simulink model "trafficLight"  (R2024a)
settings: Solver=FixedStepDiscrete  StartTime=0.0  StopTime=inf  FixedStep=1e-2  RelTol=1e-3  EnableMultiTasking=on
libraries: stm32f4xxblockslib x4
settings Model: STM32="{\"DigitalPortWrite\":[{\"ID\":\"untitled:5\"},{\"ID\":\"untitled:6\"},{\"ID\":\"untitled:7\"},{\"ID\":\"trafficLight:5\"},{\"ID\":\"trafficLight:7\"},{\"ID\":\"trafficLight:6\"}],\"HardwareInterrupt\":[{\"ID\":\"untitled:8\"},{\"ID\":\"trafficLight:8\"}]}"  Creator=User  LastModifiedBy=User
settings SolverCC: AutoInsertRateTranBlk=on
settings OptimizationCC: EnhancedBackFolding=on  PassReuseOutputArgsAs=Individual arguments  ZeroExternalMemoryAtStartup=off  ZeroInternalMemoryAtStartup=off  MaxStackSize=64  OptimizeBlockOrder=speed  DifferentSizesBufferReuse=on  OptimizationCustomize=off  EfficientTunableParamExpr=on
settings DebuggingCC: MultiTaskDSMMsg=none  ParameterTunabilityLossMsg=error
settings HardwareCC: ProdBitPerPointer=32  ProdBitPerSizeT=32  ProdBitPerPtrDiffT=32  ProdLargestAtomicInteger=Long  ProdLargestAtomicFloat=Double  ProdWordSize=32  ProdLongLongMode=on  ProdHWDeviceType=ARM Compatible->ARM Cortex-M
settings SFSimCC: MATLABDynamicMemAlloc=off
settings RTWCC: Description=Embedded Coder  SystemTargetFile=ert.tlc  HardwareBoard=STM32F4xx Based  TemplateMakefile=ert_default_tmf  Toolchain=GNU Tools for ARM Embedded Processors
settings CodeAppCC: ForceParamTrailComments=on  IgnoreCustomStorageClasses=off  OperatorAnnotations=on  SimulinkDataObjDesc=on  SFDataObjDesc=on  InsertBlockDesc=on
settings ERTTargetCC: TargetLangStandard=C99 (ISO)  CodeReplacementLibrary=ARM Cortex-M  ExtModeTransport=3  ExtModeStaticAlloc=on  ExtModeStaticAllocSize=2048  ExtModeMexFile=ext_xcp  ExtModeIntrfLevel=Level2 - Open

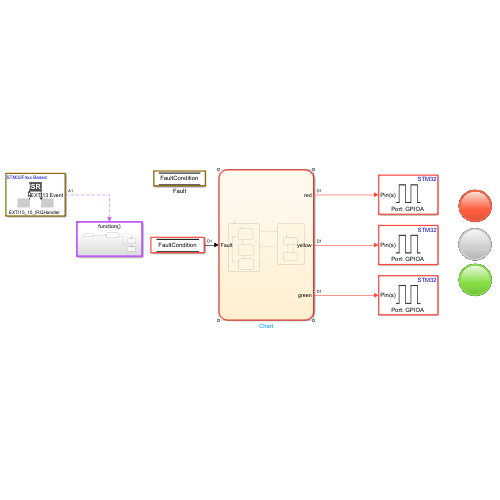
[thumbnail: Simulink's stored preview of the top-level diagram]
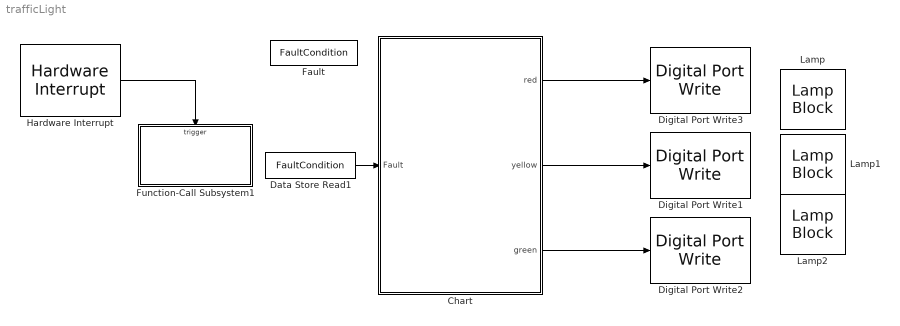
== system trafficLight ==
  Chart : Stateflow chart  TreatAsAtomicUnit=on
  Data Store Read1 : DataStoreRead  DataStoreName=FaultCondition  IndexOptions=Index vector (dialog)  Indices=1  OutputSizes=1
  Digital Port Write1 : stm32f4xxblockslib/Digital Port Write  PortName=GPIOA  PinNumber=[11]  ReadOperation=off  IOAsArray=on  EnableSimPort=off  hoistedMaskSrc=ECSoC/ECSimCodegen/Digital Port Write
  Digital Port Write2 : stm32f4xxblockslib/Digital Port Write  PortName=GPIOA  PinNumber=[12]  ReadOperation=off  IOAsArray=on  EnableSimPort=off  hoistedMaskSrc=ECSoC/ECSimCodegen/Digital Port Write
  Digital Port Write3 : stm32f4xxblockslib/Digital Port Write  PortName=GPIOA  PinNumber=[10]  ReadOperation=off  IOAsArray=on  EnableSimPort=off  hoistedMaskSrc=ECSoC/ECSimCodegen/Digital Port Write
  Fault : DataStoreMemory  DataStoreName=FaultCondition  WriteAfterWriteMsg=warning  ShowAdditionalParam=off
  Function-Call Subsystem1 : Subsystem  TreatAsAtomicUnit=on
  Hardware Interrupt : stm32f4xxblockslib/Hardware Interrupt  ISRGroup=External interrupts (EXTI)  ISRName=EXTI15_10_IRQHandler  ISRNumber=55  EventsList={ 'off', 'EXTI15 Event', '1'; 'off', 'EXTI14 Event', '2'; 'on', 'EXTI13 Event', '3'; 'off', 'EXTI12 Event', '4'; 'off', 'EXTI11 Event', '5'; 'off', 'EXTI10 Event', '6'; 'off', 'Custom event', '7' }  SelectedEvents={'EXTI13 Event'}  TaskPriority=30  DisablePreemption=on  ClearInterruptFlagsAtEndOfEvent=off  InterruptDefinitionFile=$(TARGET_ROOT)/registry/interrupts/STM32F4xxBased_interrupts.xml  HardwareBoard=STM32F4xx Based  EnableSimPort=off
  Lamp : LampBlock  LabelPosition=Hide
  Lamp1 : LampBlock  LabelPosition=Hide
  Lamp2 : LampBlock  LabelPosition=Hide
  wires:
  Chart/1(red) -> Digital Port Write3/1
  Chart/2(yellow) -> Digital Port Write1/1
  Chart/3(green) -> Digital Port Write2/1
  Hardware Interrupt/1 -> Function-Call Subsystem1/Trigger
  Data Store Read1/1 -> Chart/1(Fault)

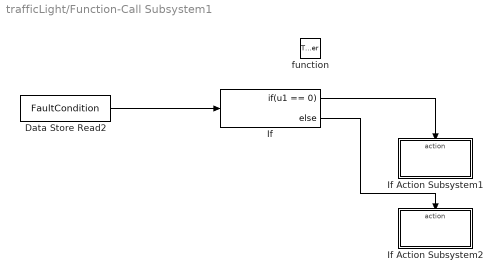
== system trafficLight/Function-Call Subsystem1 ==
  function : TriggerPort  TriggerType=function-call  VariantControl=(inherit)
  Data Store Read2 : DataStoreRead  DataStoreName=FaultCondition  IndexOptions=Index vector (dialog)  Indices=1  OutputSizes=1
  If : If  IfExpression=u1 == 0
  If Action Subsystem1 : Subsystem  TreatAsAtomicUnit=on
  If Action Subsystem2 : Subsystem  TreatAsAtomicUnit=on
  wires:
  If/1 -> If Action Subsystem1/Action
  Data Store Read2/1 -> If/1
  If/2 -> If Action Subsystem2/Action

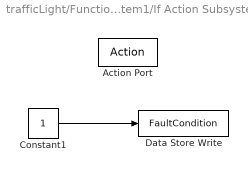
== system trafficLight/Function-Call Subsystem1/If Action Subsystem1 ==
  Action Port : ActionPort  ActionPortLabel=if(u1 == 0)
  Constant1 : Constant  OutDataTypeStr=boolean
  Data Store Write : DataStoreWrite  DataStoreName=FaultCondition  IndexOptions=Index vector (dialog)  Indices=1  OutputSizes=1
  wires:
  Constant1/1 -> Data Store Write/1

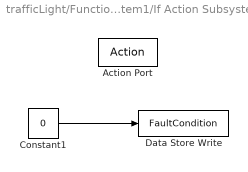
== system trafficLight/Function-Call Subsystem1/If Action Subsystem2 ==
  Action Port : ActionPort  ActionPortLabel=else
  Constant1 : Constant  Value=0  OutDataTypeStr=boolean
  Data Store Write : DataStoreWrite  DataStoreName=FaultCondition  IndexOptions=Index vector (dialog)  Indices=1  OutputSizes=1
  wires:
  Constant1/1 -> Data Store Write/1

== stateflow chart trafficLight/Chart ==
  state Normal
    (history)
    state Stop
      % Red light
      entry:
      red = 1;
      yellow = 0;
      green = 0;
    state PrepareToStop
      % Yellow light
      entry:
      red = 0;
      yellow = 1;
      green = 0;
    state Go
      % Green light
      entry:
      red = 0;
      yellow = 0;
      green = 1;
    (default) -> Stop
    Stop -> (junction 35)
    (junction 35) -> (junction 43) : after(2,sec)
    PrepareToStop -> Stop : after(2,sec)
    Go -> PrepareToStop : after(2,sec)
    (junction 43) -> Go
  state Fault
    entry:
    yellow = 0;
    green = 0;
    state BlinkOn
      % Red light
      entry:
      red = 1;
    state BlinkOff
      % No light
      entry:
      red = 0;
    (default) -> BlinkOn
    BlinkOff -> BlinkOn : after(1,sec)
    BlinkOn -> BlinkOff : after(1,sec)
  (default) -> Normal
  Normal -> Fault : [Fault  == 1]
  Fault -> Normal : [Fault == 0]
  data: red output boolean; yellow output boolean; green output boolean; Fault input boolean
